simulink model "RoverSim"  (R2024b)
settings: Solver=FixedStepAuto  StartTime=0.0  StopTime=30  FixedStep=0.5  RelTol=1e-3
values from neighbouring files (symbols this model uses):
  env = Environment()    [Main.m]
libraries: slpidlib x2
settings Model: Creator=Psychlone  LastModifiedBy=Psychlone

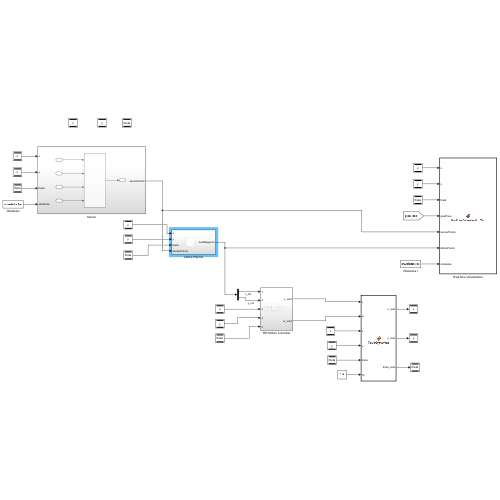
[thumbnail: Simulink's stored preview of the top-level diagram]
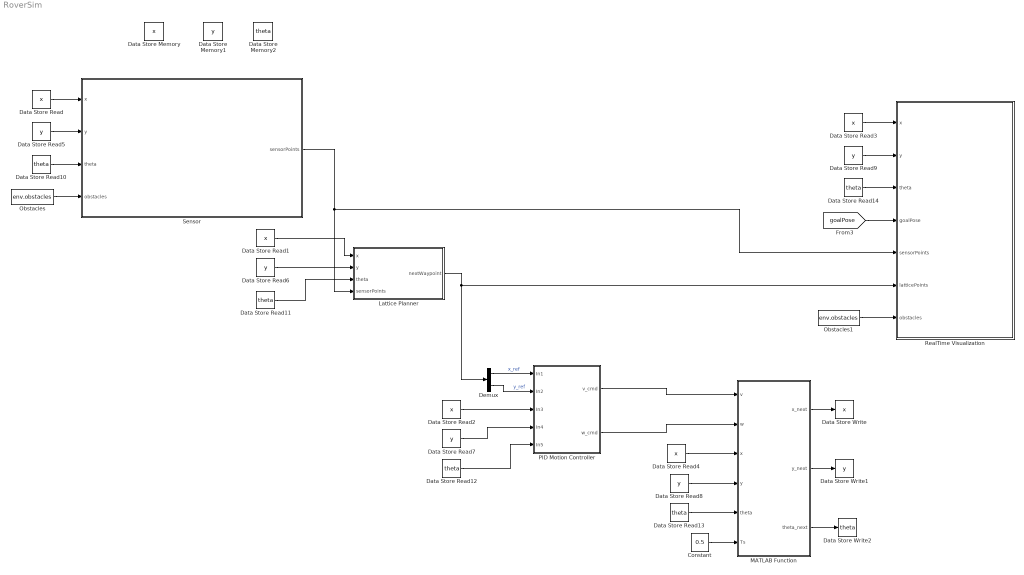
== system RoverSim ==
  Constant : Constant  Value=0.5
  Data Store Memory : DataStoreMemory  DataStoreName=x  WriteAfterWriteMsg=warning  InitialValue=env.startPose(1)  ShowAdditionalParam=off
  Data Store Memory1 : DataStoreMemory  DataStoreName=y  WriteAfterWriteMsg=warning  InitialValue=env.startPose(2)  ShowAdditionalParam=off
  Data Store Memory2 : DataStoreMemory  DataStoreName=theta  WriteAfterWriteMsg=warning  InitialValue=env.startPose(3)  ShowAdditionalParam=off
  Data Store Read{,1..4} (5 alike) : DataStoreRead  DataStoreName=x  IndexOptions=Index vector (dialog)  Indices=1  OutputSizes=1
  Data Store Read{10..14} (5 alike) : DataStoreRead  DataStoreName=theta  IndexOptions=Index vector (dialog)  Indices=1  OutputSizes=1
  Data Store Read{5..9} (5 alike) : DataStoreRead  DataStoreName=y  IndexOptions=Index vector (dialog)  Indices=1  OutputSizes=1
  Data Store Write : DataStoreWrite  DataStoreName=x  IndexOptions=Index vector (dialog)  Indices=1  OutputSizes=1
  Data Store Write1 : DataStoreWrite  DataStoreName=y  IndexOptions=Index vector (dialog)  Indices=1  OutputSizes=1
  Data Store Write2 : DataStoreWrite  DataStoreName=theta  IndexOptions=Index vector (dialog)  Indices=1  OutputSizes=1
  Demux : Demux  Outputs=2
  Lattice Planner : Subsystem  Priority=2
  MATLAB Function : MATLAB Function  Priority=4  TreatAsAtomicUnit=on
  Obstacles : Constant  Value=env.obstacles
  Obstacles1 : Constant  Value=env.obstacles
  PID Motion Controller : Subsystem  Priority=3
  RealTime Visualization : MATLAB Function  Priority=5  TreatAsAtomicUnit=on
  Sensor : Subsystem  Priority=1
  wires:
  Sensor/1(sensorPoints) -> Lattice Planner/4(sensorPoints), RealTime Visualization/5(sensorPoints)
  Lattice Planner/1(nextWaypoint) -> Demux/1, RealTime Visualization/6(latticePoints)
  Demux/1 -> PID Motion Controller/1(In1)  "x_ref"
  Demux/2 -> PID Motion Controller/2(In2)  "y_ref"
  Data Store Read3/1 -> RealTime Visualization/1(x)
  Data Store Read9/1 -> RealTime Visualization/2(y)
  Data Store Read14/1 -> RealTime Visualization/3(theta)
  [goalPose] -> RealTime Visualization/4(goalPose)
  Data Store Read1/1 -> Lattice Planner/1(x)
  Data Store Read6/1 -> Lattice Planner/2(y)
  Data Store Read11/1 -> Lattice Planner/3(theta)
  Data Store Read2/1 -> PID Motion Controller/3(In3)
  Data Store Read7/1 -> PID Motion Controller/4(In4)
  Data Store Read12/1 -> PID Motion Controller/5(In5)
  Data Store Read/1 -> Sensor/1(x)
  Data Store Read5/1 -> Sensor/2(y)
  Data Store Read10/1 -> Sensor/3(theta)
  PID Motion Controller/1(v_cmd) -> MATLAB Function/1(v)
  PID Motion Controller/2(w_cmd) -> MATLAB Function/2(w)
  Constant/1 -> MATLAB Function/6(Ts)
  Data Store Read4/1 -> MATLAB Function/3(x)
  Data Store Read8/1 -> MATLAB Function/4(y)
  Data Store Read13/1 -> MATLAB Function/5(theta)
  Obstacles/1 -> Sensor/4(obstacles)
  Obstacles1/1 -> RealTime Visualization/7(obstacles)
  MATLAB Function/3(theta_next) -> Data Store Write2/1
  MATLAB Function/2(y_next) -> Data Store Write1/1
  MATLAB Function/1(x_next) -> Data Store Write/1

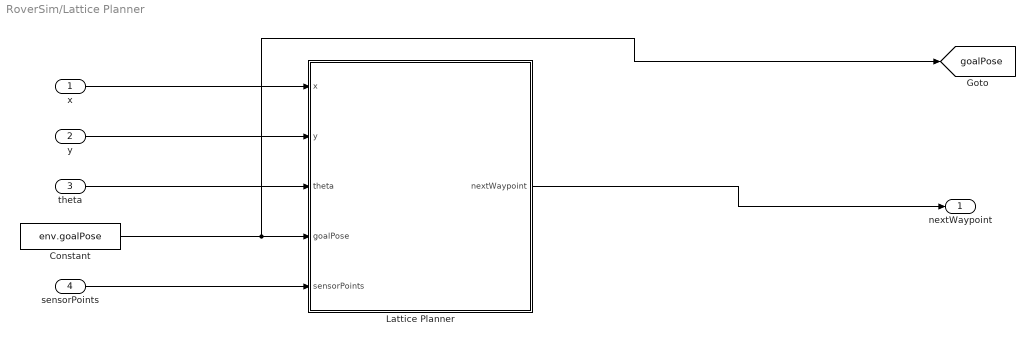
== system RoverSim/Lattice Planner ==
  x : Inport
  y : Inport  Port=2
  theta : Inport  Port=3
  sensorPoints : Inport  Port=4
  Constant : Constant  Value=env.goalPose
  Lattice Planner : MATLAB Function  TreatAsAtomicUnit=on
  nextWaypoint : Outport
  tag scope: goalPose=global
  wires:
  theta/1 -> Lattice Planner/3(theta)
  Constant/1 -> [goalPose], Lattice Planner/4(goalPose)
  x/1 -> Lattice Planner/1(x)
  sensorPoints/1 -> Lattice Planner/5(sensorPoints)
  y/1 -> Lattice Planner/2(y)
  Lattice Planner/1(nextWaypoint) -> nextWaypoint/1

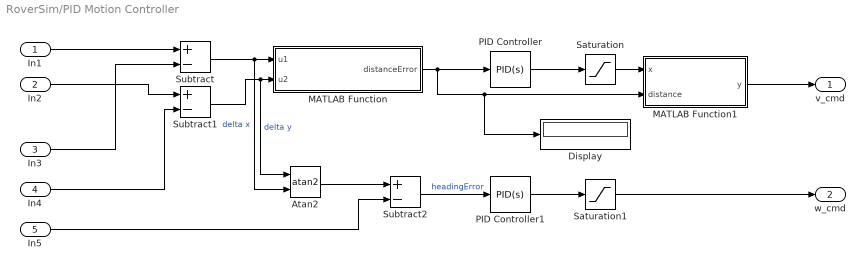
== system RoverSim/PID Motion Controller ==
  In1 : Inport
  In2 : Inport  Port=2
  In3 : Inport  Port=3
  In4 : Inport  Port=4
  In5 : Inport  Port=5
  Atan2 : Trigonometry  Operator=atan2
  Display : Display
  MATLAB Function : MATLAB Function  TreatAsAtomicUnit=on
  MATLAB Function1 : MATLAB Function  TreatAsAtomicUnit=on
  PID Controller : slpidlib/PID Controller  Controller=PID  Form=Parallel  TimeDomain=Continuous-time  UseExternalTs=off  SampleTime=-1  IntegratorMethod=Forward Euler  FilterMethod=Forward Euler  ControllerParametersSource=internal  P=1  I=0  UseKiTs=off  D=0  UseExternalDerivativeSource=off  N=100  UseFilter=on  TunerSelectOption=Transfer Function Based (PID Tuner App)  InitialConditionSource=internal  InitialConditionForIntegrator=0  InitialConditionForFilter=0  DifferentiatorICPrevScaledInput=0  ExternalReset=none  TrackingMode=off  Kt=1  LimitOutput=off  SatLimitsSource=internal  UpperSaturationLimit=inf  LowerSaturationLimit=-inf  LinearizeAsGain=on  AntiWindupMode=none  Kb=1  LimitIntegrator=off  UpperIntegratorSaturationLimit=inf  LowerIntegratorSaturationLimit=-inf  POutMin=[]  POutMax=[]  IOutMin=[]  IOutMax=[]  DOutMin=[]  DOutMax=[]  NOutMin=[]  NOutMax=[]  SumOutMin=[]  SumOutMax=[]  SaturationOutMin=[]  SaturationOutMax=[]  PParamMin=[]  PParamMax=[]  IParamMin=[]  IParamMax=[]  DParamMin=[]  DParamMax=[]  NParamMin=[]  NParamMax=[]  KbParamMin=[]  KbParamMax=[]  KtParamMin=[]  KtParamMax=[]  KbOutMin=[]  KbOutMax=[]  KtOutMin=[]  KtOutMax=[]  IntegratorOutMin=[]  IntegratorOutMax=[]  FilterOutMin=[]  FilterOutMax=[]  SumI1OutMin=[]  SumI1OutMax=[]  SumI2OutMin=[]  SumI2OutMax=[]  SumI3OutMin=[]  SumI3OutMax=[]  SumI4OutMin=[]  SumI4OutMax=[]  SumDOutMin=[]  SumDOutMax=[]  DifferentiatorOutMin=[]  DifferentiatorOutMax=[]  FilterDiffOutCoefMin=[]  FilterDiffOutCoefMax=[]  ReciprocalOutMin=[]  ReciprocalOutMax=[]  SumDenOutMin=[]  SumDenOutMax=[]  SumNumOutMin=[]  SumNumOutMax=[]  DivideOutMin=[]  DivideOutMax=[]  UdiffTsProdOutMin=[]  UdiffTsProdOutMax=[]  NTsProdOutMin=[]  NTsProdOutMax=[]  UintegralTsProdOutMin=[]  UintegralTsProdOutMax=[]  UngainTsProdOutMin=[]  UngainTsProdOutMax=[]  ClampingZeroOutDataTypeStr=Inherit: Inherit via back propagation  ClampingZeroOutMin=[]  ClampingZeroOutMax=[]  FilterDenConstantOutDataTypeStr=Inherit: Inherit via back propagation  FilterDenConstantOutMin=[]  FilterDenConstantOutMax=[]  PCopyOutDataTypeStr=Inherit: Inherit via back propagation  PCopyOutMin=[]  PCopyOutMax=[]  NCopyOutDataTypeStr=Inherit: Inherit via back propagation  NCopyOutMin=[]  NCopyOutMax=[]  IntegratorContinuousStateAttributes=''  IntegratorStateMustResolveToSignalObject=off  IntegratorRTWStateStorageClass=Auto  FilterContinuousStateAttributes=''  FilterStateMustResolveToSignalObject=off  FilterRTWStateStorageClass=Auto  ParallelPVariant=InternalParameters  IdealPVariant=Disabled  IVariant=InternalParameters  DVariant=InternalParameters  IntegratorVariant=Continuous  SatVariant=Disabled  AWVariant=Passthrough  PCopyVariant=Disabled  TRVariant=Disabled  FdbkBlocksVariant=Forward  IdealPFdbkVariant=Disabled  SatFdbkVariant=Disabled  DerivativeFilterVariant=ContFilter  NVariant=InternalParameters  NCopyVariant=Disabled  FilterICVariant=InternalICsFilter  IntegratorICVariant=InternalICs  ExternalResetVariant=Disabled  TRSumVariant=Passthrough  SumFdbkVariant=Disabled  SumVariant=Sum_PID  TsampFilterVariant=InternalTs  TsampNgainVariant=Passthrough  TsampIntegralVariant=Disabled_SignalSpec  ExternalSaturationOutDataTypeStr=Inherit: Same as second input  DerivativeSourceVariant=ErrorSignal  PreIntVariant=InternalPreInt
  PID Controller1 : slpidlib/PID Controller  Controller=PID  Form=Parallel  TimeDomain=Continuous-time  UseExternalTs=off  SampleTime=-1  IntegratorMethod=Forward Euler  FilterMethod=Forward Euler  ControllerParametersSource=internal  P=2  I=0  UseKiTs=off  D=0.2  UseExternalDerivativeSource=off  N=100  UseFilter=on  TunerSelectOption=Transfer Function Based (PID Tuner App)  InitialConditionSource=internal  InitialConditionForIntegrator=0  InitialConditionForFilter=0  DifferentiatorICPrevScaledInput=0  ExternalReset=none  TrackingMode=off  Kt=1  LimitOutput=off  SatLimitsSource=internal  UpperSaturationLimit=inf  LowerSaturationLimit=-inf  LinearizeAsGain=on  AntiWindupMode=none  Kb=1  LimitIntegrator=off  UpperIntegratorSaturationLimit=inf  LowerIntegratorSaturationLimit=-inf  POutMin=[]  POutMax=[]  IOutMin=[]  IOutMax=[]  DOutMin=[]  DOutMax=[]  NOutMin=[]  NOutMax=[]  SumOutMin=[]  SumOutMax=[]  SaturationOutMin=[]  SaturationOutMax=[]  PParamMin=[]  PParamMax=[]  IParamMin=[]  IParamMax=[]  DParamMin=[]  DParamMax=[]  NParamMin=[]  NParamMax=[]  KbParamMin=[]  KbParamMax=[]  KtParamMin=[]  KtParamMax=[]  KbOutMin=[]  KbOutMax=[]  KtOutMin=[]  KtOutMax=[]  IntegratorOutMin=[]  IntegratorOutMax=[]  FilterOutMin=[]  FilterOutMax=[]  SumI1OutMin=[]  SumI1OutMax=[]  SumI2OutMin=[]  SumI2OutMax=[]  SumI3OutMin=[]  SumI3OutMax=[]  SumI4OutMin=[]  SumI4OutMax=[]  SumDOutMin=[]  SumDOutMax=[]  DifferentiatorOutMin=[]  DifferentiatorOutMax=[]  FilterDiffOutCoefMin=[]  FilterDiffOutCoefMax=[]  ReciprocalOutMin=[]  ReciprocalOutMax=[]  SumDenOutMin=[]  SumDenOutMax=[]  SumNumOutMin=[]  SumNumOutMax=[]  DivideOutMin=[]  DivideOutMax=[]  UdiffTsProdOutMin=[]  UdiffTsProdOutMax=[]  NTsProdOutMin=[]  NTsProdOutMax=[]  UintegralTsProdOutMin=[]  UintegralTsProdOutMax=[]  UngainTsProdOutMin=[]  UngainTsProdOutMax=[]  ClampingZeroOutDataTypeStr=Inherit: Inherit via back propagation  ClampingZeroOutMin=[]  ClampingZeroOutMax=[]  FilterDenConstantOutDataTypeStr=Inherit: Inherit via back propagation  FilterDenConstantOutMin=[]  FilterDenConstantOutMax=[]  PCopyOutDataTypeStr=Inherit: Inherit via back propagation  PCopyOutMin=[]  PCopyOutMax=[]  NCopyOutDataTypeStr=Inherit: Inherit via back propagation  NCopyOutMin=[]  NCopyOutMax=[]  IntegratorContinuousStateAttributes=''  IntegratorStateMustResolveToSignalObject=off  IntegratorRTWStateStorageClass=Auto  FilterContinuousStateAttributes=''  FilterStateMustResolveToSignalObject=off  FilterRTWStateStorageClass=Auto  ParallelPVariant=InternalParameters  IdealPVariant=Disabled  IVariant=InternalParameters  DVariant=InternalParameters  IntegratorVariant=Continuous  SatVariant=Disabled  AWVariant=Passthrough  PCopyVariant=Disabled  TRVariant=Disabled  FdbkBlocksVariant=Forward  IdealPFdbkVariant=Disabled  SatFdbkVariant=Disabled  DerivativeFilterVariant=ContFilter  NVariant=InternalParameters  NCopyVariant=Disabled  FilterICVariant=InternalICsFilter  IntegratorICVariant=InternalICs  ExternalResetVariant=Disabled  TRSumVariant=Passthrough  SumFdbkVariant=Disabled  SumVariant=Sum_PID  TsampFilterVariant=InternalTs  TsampNgainVariant=Passthrough  TsampIntegralVariant=Disabled_SignalSpec  ExternalSaturationOutDataTypeStr=Inherit: Same as second input  DerivativeSourceVariant=ErrorSignal  PreIntVariant=InternalPreInt
  Saturation : Saturate  UpperLimit=1  LowerLimit=0
  Saturation1 : Saturate  UpperLimit=2  LowerLimit=-2
  Subtract : Sum  Inputs=+-
  Subtract1 : Sum  Inputs=+-
  Subtract2 : Sum  Inputs=+-
  v_cmd : Outport
  w_cmd : Outport  Port=2
  wires:
  In1/1 -> Subtract/1
  In3/1 -> Subtract/2
  In2/1 -> Subtract1/1
  In4/1 -> Subtract1/2
  Subtract/1 -> Atan2/2, MATLAB Function/1(u1)  "delta x"
  Subtract1/1 -> Atan2/1, MATLAB Function/2(u2)  "delta y"
  MATLAB Function/1(distanceError) -> Display/1, MATLAB Function1/2(distance), PID Controller/1
  Atan2/1 -> Subtract2/1
  In5/1 -> Subtract2/2
  Subtract2/1 -> PID Controller1/1  "headingError"
  PID Controller/1 -> Saturation/1
  Saturation1/1 -> w_cmd/1
  PID Controller1/1 -> Saturation1/1
  Saturation/1 -> MATLAB Function1/1(x)
  MATLAB Function1/1(y) -> v_cmd/1

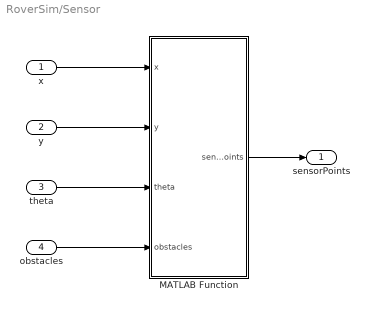
== system RoverSim/Sensor ==
  x : Inport
  y : Inport  Port=2
  theta : Inport  Port=3
  obstacles : Inport  Port=4
  MATLAB Function : MATLAB Function  TreatAsAtomicUnit=on
  sensorPoints : Outport
  wires:
  MATLAB Function/1(sensorPoints) -> sensorPoints/1
  x/1 -> MATLAB Function/1(x)
  y/1 -> MATLAB Function/2(y)
  theta/1 -> MATLAB Function/3(theta)
  obstacles/1 -> MATLAB Function/4(obstacles)

== matlab function RoverSim/Lattice Planner/Lattice Planner ==
  data: x input; nextWaypoint output; y input; theta input; goalPose input; sensorPoints input
function nextWaypoint = GoalHeadingAvoid(x, y, theta, goalPose, sensorPoints)
%#codegen
% +Y-forward rover frame:
%   - sensorPoints are in rover frame: [xR (right), yR (forward)]

%% Tunables
stepLen        = 0.6;     % length of each step (m)
corrHalfWidth  = 0.30;    % half-width of forward corridor (m)
forwardMargin  = 0.05;    % extra corridor length (m)
avoidAngle     = deg2rad(25); % turn-away angle when blocked
maxTries       = 3;       % try a few larger deviations if still blocked

%% 0) sensor points (NaN rows -> remove)
if isempty(sensorPoints)
    pts = zeros(0,2);
else
    mask = ~any(isnan(sensorPoints),2);
    pts  = sensorPoints(mask,:);
end

%% 1) Goal direction in ROVER frame (angle from +Y-forward)
% World -> rover transform for a vector [dx;dy] with +Y forward, +X right:

dxg = goalPose(1) - x;
dyg = goalPose(2) - y;
if dxg == 0 && dyg == 0
    nextWaypoint = [x, y];  % already at goal
    return;
end
xRg =  sin(theta)*dxg - cos(theta)*dyg;   % lateral in rover frame (right +)
yRg =  cos(theta)*dxg + sin(theta)*dyg;   % forward in rover frame
goalAng = atan2(xRg, yRg);                % angle from +Y (forward). 0 = straight ahead

%% 2) Corridor check helper

function free = corridorClear(phi)
    if isempty(pts)
        free = true; return;
    end
    c = cos(phi); s = sin(phi);
    xC =  c*pts(:,1) + s*pts(:,2);
    yC = -s*pts(:,1) + c*pts(:,2);
    inY = (yC > 0) & (yC < (stepLen + forwardMargin));
    inX = abs(xC) <= corrHalfWidth;
    free = ~any(inY & inX);
end

%% 3) Try straight-to-goal first; if blocked, steer away from nearest obstacle
phi = goalAng;

if ~corridorClear(phi)
    % Find nearest obstacle AHEAD (yR > 0)
    aheadMask = ~isempty(pts) & (pts(:,2) > 0);
    if any(aheadMask)
        aheadPts = pts(aheadMask,:);
        d2 = aheadPts(:,1).^2 + aheadPts(:,2).^2;
        [~,iMin] = min(d2);
        xR_near = aheadPts(iMin,1);   % lateral: right(+), left(-)
        % Turn away from obstacle (if obstacle on right, steer left, i.e., negative x)
        steerSign = -sign(xR_near);   % left if +xR, right if -xR; if 0, steer left
        if steerSign == 0, steerSign = 1; end

        % Try a few increasing deviations
        tried = false;
        for k = 1:maxTries
            phiTry = phi + steerSign * (k * avoidAngle);
            if corridorClear(phiTry)
                phi = phiTry;
                tried = true;
                break;
            end
        end
        % If still blocked, try the other side
        if ~tried
            for k = 1:maxTries
                phiTry = phi - steerSign * (k * avoidAngle);
                if corridorClear(phiTry)
                    phi = phiTry;
                    tried = true;
                    break;
                end
            end
        end
        % If still blocked, fall through with original phi (we'll take a small nudge)
    end
end

%% 4) Produce the waypoint in WORLD frame

xR_step = stepLen * sin(phi);
yR_step = stepLen * cos(phi);
dx =  sin(theta)*xR_step + cos(theta)*yR_step;
dy = -cos(theta)*xR_step + sin(theta)*yR_step;

% If corridor is utterly blocked, make a tiny nudge forward to avoid deadlock
if ~corridorClear(phi)
    dx = 0.25 * cos(theta);   % small forward nudge in world (approx)
    dy = 0.25 * sin(theta);
end

nextWaypoint = [x + dx, y + dy];
end

== matlab function RoverSim/Sensor/MATLAB Function ==
  data: x input; sensorPoints output; y input; theta input; obstacles input
function sensorPoints = SensorsBlock(x, y, theta, obstacles)
%#codegen
% Inputs:
%   x, y, theta  - rover pose in world frame
%   obstacles    - Nx4 array [x_center, y_center, width, height]
% Output:
%   sensorPoints - Nx2 array of points (in rover frame)

%% Sensor parameters
FOV = deg2rad(120);     % 120° horizontal FOV
rangeMax = 10;          % max range (m)
pointSpacing = 0.2;     % sampling grid for obstacle points
maxPoints = 5000;       % safety cap
sensorPoints = nan(maxPoints,2); 
count = 0;

%% Loop through all obstacles
for i = 1:size(obstacles,1)
    obs = obstacles(i,:);
    xMin = obs(1) - obs(3)/2;
    xMax = obs(1) + obs(3)/2;
    yMin = obs(2) - obs(4)/2;
    yMax = obs(2) + obs(4)/2;

    % Generate a grid of obstacle surface points
    xVec = xMin:pointSpacing:xMax;
    yVec = yMin:pointSpacing:yMax;
    
    for xi = 1:length(xVec)
        for yi = 1:length(yVec)
            px = xVec(xi);
            py = yVec(yi);

            % Vector from rover to obstacle in world coordinates
            dx = px - x;
            dy = py - y;

            % Transform world → rover frame (inverse rotation)
            % Rover's local +X = forward, +Y = left
            xR =  sin(theta)*dx - cos(theta)*dy;  % right (+) / left (-)
            yR =  cos(theta)*dx + sin(theta)*dy;  % forward (+)

            % Only consider points within range and in front of rover
            dist_sq = xR^2 + yR^2;
            if (yR > 0) && (dist_sq <= rangeMax^2)
                angle = atan2(xR, yR);  % now angle measured from forward (+Y)
                if abs(angle) <= FOV/2
                    count = count + 1;
                    if count <= maxPoints
                        sensorPoints(count,:) = [xR, yR];
                    end
                end
            end
        end
    end
end

end

== matlab function RoverSim/RealTime Visualization ==
  data: x input; y input; theta input; goalPose input; sensorPoints input; latticePoints input; obstacles input
function RealTimeVisualizationSim(x, y, theta, goalPose, sensorPoints, latticePoints, obstacles)
%#codegen
persistent figHandle isInitialized
if isempty(isInitialized)
    figHandle = figure('Name','Rover Real-Time Visualization');
    isInitialized = true;
end

figure(figHandle);
clf(figHandle); hold on; grid on; axis equal;
xlabel('X [m]'); ylabel('Y [m]');
title('Rover Local Lattice & Sensor Visualization');

%% Obstacles
for i = 1:size(obstacles,1)
    obs = obstacles(i,:);
    rectangle('Position',[obs(1)-obs(3)/2, obs(2)-obs(4)/2, obs(3), obs(4)],...
              'FaceColor',[0.8 0.1 0.1 0.5],'EdgeColor','k');
end

%% Rover body
bodyL = 0.3; bodyW = 0.5;
corners = [ bodyL/2  bodyW/2;
            bodyL/2 -bodyW/2;
           -bodyL/2 -bodyW/2;
           -bodyL/2  bodyW/2;
            bodyL/2  bodyW/2]';
Rbody = [cos(theta) -sin(theta); sin(theta) cos(theta)];
bodyXY = Rbody * corners + [x; y];
plot(bodyXY(1,:), bodyXY(2,:), 'b-', 'LineWidth', 1.5, 'DisplayName','Rover Body');

%% Camera FOV
FOV = deg2rad(120); rangeMax = 10;
angles = linspace(-FOV/2, FOV/2, 30);
fovX_local = [0, rangeMax*cos(angles)];
fovY_local = [0, rangeMax*sin(angles)];
Rfov = [cos(theta) -sin(theta); sin(theta) cos(theta)];
fovWorld = Rfov * [fovX_local; fovY_local] + [x; y];
fill([x fovWorld(1,:)],[y fovWorld(2,:)],'c','FaceAlpha',0.1,'EdgeColor','c','DisplayName','Camera FOV');

%% Sensor points (rover frame → world)
if ~isempty(sensorPoints) && ~all(isnan(sensorPoints(:)))
    sensorPoints = sensorPoints(~any(isnan(sensorPoints),2), :);
    % rover → world (match +Y forward convention)
    R = [ sin(theta)  cos(theta);
         -cos(theta)  sin(theta) ];
    sensorWorld = (R * sensorPoints' + [x; y])';

    plot(sensorWorld(:,1), sensorWorld(:,2),'g.','MarkerSize',8,'DisplayName','Sensor Points');
end

%% Lattice points
if ~isempty(latticePoints) && ~all(isnan(latticePoints(:)))
    latticePoints = latticePoints(~any(isnan(latticePoints),2), :);
    plot(latticePoints(:,1), latticePoints(:,2),'mo','MarkerFaceColor','m','DisplayName','Lattice Points');
end

%% Rover pose & heading
plot(x, y, 'bo','MarkerFaceColor','b','MarkerSize',10,'DisplayName','Rover Position');
quiver(x, y, cos(theta), sin(theta), 0.5,'b','LineWidth',1.5);

%% Goal
plot(goalPose(1), goalPose(2), 'ro','MarkerFaceColor','r','MarkerSize',10,'DisplayName','Goal');

legend('Location','bestoutside');
drawnow;
end

== matlab function RoverSim/PID Motion Controller/MATLAB Function ==
  data: u1 input; distanceError output; u2 input
function distanceError = fcn(u1,u2)
distanceError = sqrt(u1^2 + u2^2);
end

== matlab function RoverSim/PID Motion Controller/MATLAB Function1 ==
  data: x input; y output; distance input
function y = fcn(x,distance)

switch distance
    case 0 
        y= 0;
    case 0.1
        y= 0;
    otherwise
        y=x;
end

== matlab function RoverSim/MATLAB Function ==
  data: v input; x_next output; w input; x input; y input; theta input; Ts input; y_next output; theta_next output
function [x_next, y_next, theta_next] = RoverDynamics(v, w, x, y, theta, Ts)
%#codegen
% Simple kinematic unicycle model for rover dynamics

% Integrate kinematics (Euler method)
x_next     = x + Ts * v * cos(theta);
y_next     = y + Ts * v * sin(theta);
theta_next = theta + Ts * w;

% Normalize angle to [-pi, pi]
theta_next = atan2(sin(theta_next), cos(theta_next));

end
